simulink model "Rex_ProblemSet_4"  (R2020a)
settings: Solver=VariableStepAuto  StartTime=0.0  StopTime=10.0  RelTol=1e-3
libraries: commutil2 x4
settings Model: Creator=bayntuna  LastModifiedBy=23RexL

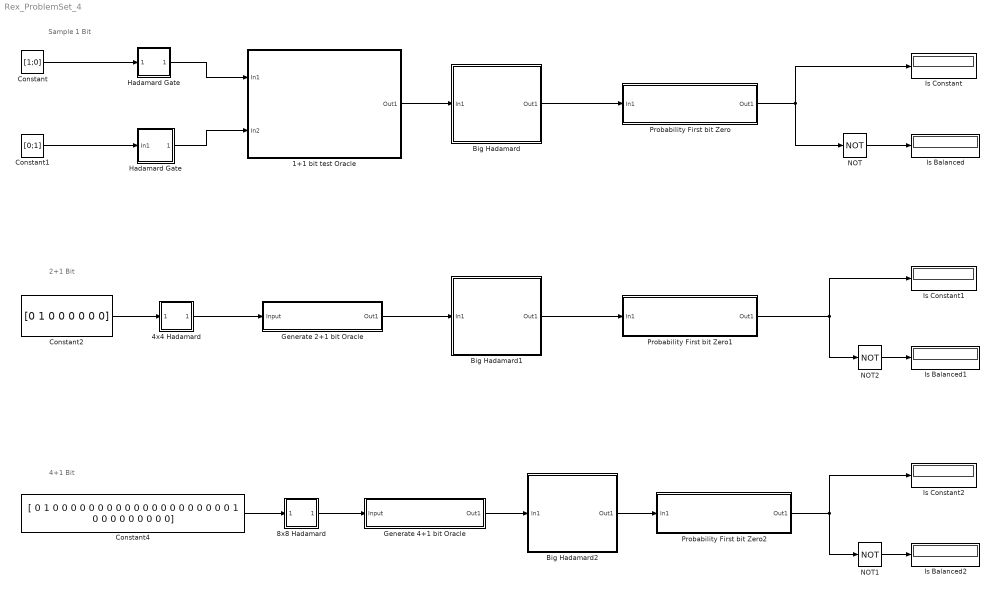
== system Rex_ProblemSet_4 ==
  note: 4+1 Bit
  note: 2+1 Bit
  note: Sample 1 Bit
  1+1 bit test Oracle : Subsystem
  4x4 Hadamard : Subsystem
  8x8 Hadamard : Subsystem
  Big Hadamard : Subsystem
  Big Hadamard1 : Subsystem
  Big Hadamard2 : Subsystem
  Constant : Constant  Value=[1;0]
  Constant1 : Constant  Value=[0;1]
  Constant2 : Constant  Value=[0 1 0 0 0 0 0 0]
  Constant4 : Constant  Value=[ 0 1 0 0 0 0 0 0 0 0 0 0 0 0 0 0 0 0 0 0 0 0 1 0 0 0 0 0 0 0 0 0]
  Generate 2+1 bit Oracle : Subsystem
  Generate 4+1 bit Oracle : Subsystem
  Hadamard Gate : Subsystem
  "Hadamard Gate " : Subsystem
  Is Balanced : Display
  Is Balanced1 : Display
  Is Balanced2 : Display
  Is Constant : Display
  Is Constant1 : Display
  Is Constant2 : Display
  NOT : Logic  Operator=NOT  IconShape=distinctive  AllPortsSameDT=off  OutDataTypeStr=boolean
  NOT1 : Logic  Operator=NOT  IconShape=distinctive  AllPortsSameDT=off  OutDataTypeStr=boolean
  NOT2 : Logic  Operator=NOT  IconShape=distinctive  AllPortsSameDT=off  OutDataTypeStr=boolean
  Probability First bit Zero : Subsystem
  Probability First bit Zero1 : Subsystem
  Probability First bit Zero2 : Subsystem
  wires:
  Constant/1 -> "Hadamard Gate "/1(In1)
  Constant1/1 -> Hadamard Gate/1(In1)
  "Hadamard Gate "/1(Out1) -> 1+1 bit test Oracle/1(In1)
  Hadamard Gate/1(Out1) -> 1+1 bit test Oracle/2(In2)
  1+1 bit test Oracle/1(Out1) -> Big Hadamard/1(In1)
  Big Hadamard/1(Out1) -> Probability First bit Zero/1(In1)
  Probability First bit Zero/1(Out1) -> Is Constant/1, NOT/1
  NOT/1 -> Is Balanced/1
  Generate 2+1 bit Oracle/1(Out1) -> Big Hadamard1/1(In1)
  NOT2/1 -> Is Balanced1/1
  Probability First bit Zero1/1(Out1) -> Is Constant1/1, NOT2/1
  Big Hadamard1/1(Out1) -> Probability First bit Zero1/1(In1)
  4x4 Hadamard/1(Input) -> Generate 2+1 bit Oracle/1(Input)
  Constant2/1 -> 4x4 Hadamard/1(In1)
  Constant4/1 -> 8x8 Hadamard/1(In1)
  8x8 Hadamard/1(Input) -> Generate 4+1 bit Oracle/1(Input)
  Generate 4+1 bit Oracle/1(Out1) -> Big Hadamard2/1(In1)
  Probability First bit Zero2/1(Out1) -> Is Constant2/1, NOT1/1
  NOT1/1 -> Is Balanced2/1
  Big Hadamard2/1(Out1) -> Probability First bit Zero2/1(In1)

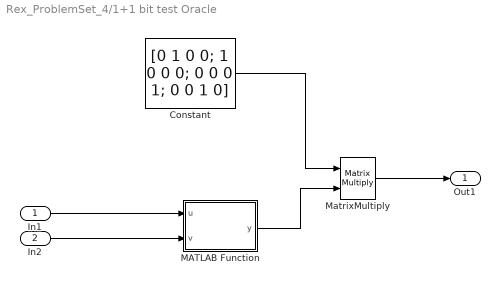
== system Rex_ProblemSet_4/1+1 bit test Oracle ==
  In1 : Inport
  In2 : Inport  Port=2
  Constant : Constant  Value=[0 1 0 0; 1 0 0 0; 0 0 0 1; 0 0 1 0]
  MATLAB Function : MATLAB Function  TreatAsAtomicUnit=on
  MatrixMultiply : Product  Multiplication=Matrix(*)
  Out1 : Outport
  wires:
  MatrixMultiply/1 -> Out1/1
  MATLAB Function/1(y) -> MatrixMultiply/2
  Constant/1 -> MatrixMultiply/1
  In1/1 -> MATLAB Function/1(u)
  In2/1 -> MATLAB Function/2(v)

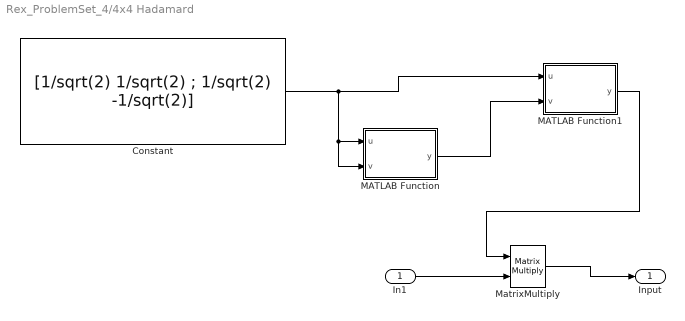
== system Rex_ProblemSet_4/4x4 Hadamard ==
  In1 : Inport
  Constant : Constant  Value=[1/sqrt(2) 1/sqrt(2) ; 1/sqrt(2) -1/sqrt(2)]
  MATLAB Function : MATLAB Function  TreatAsAtomicUnit=on
  MATLAB Function1 : MATLAB Function  TreatAsAtomicUnit=on
  MatrixMultiply : Product  Multiplication=Matrix(*)
  Input : Outport
  wires:
  MatrixMultiply/1 -> Input/1
  In1/1 -> MatrixMultiply/2
  Constant/1 -> MATLAB Function/2(v), MATLAB Function/1(u), MATLAB Function1/1(u)
  MATLAB Function/1(y) -> MATLAB Function1/2(v)
  MATLAB Function1/1(y) -> MatrixMultiply/1

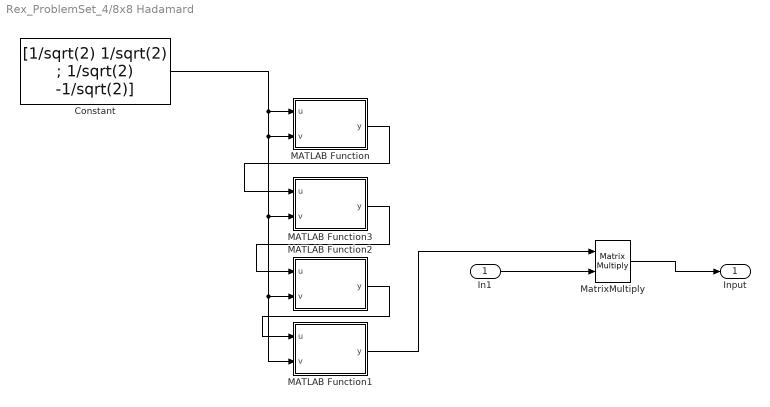
== system Rex_ProblemSet_4/8x8 Hadamard ==
  In1 : Inport
  Constant : Constant  Value=[1/sqrt(2) 1/sqrt(2) ; 1/sqrt(2) -1/sqrt(2)]
  MATLAB Function : MATLAB Function  TreatAsAtomicUnit=on
  MATLAB Function1 : MATLAB Function  TreatAsAtomicUnit=on
  MATLAB Function2 : MATLAB Function  TreatAsAtomicUnit=on
  MATLAB Function3 : MATLAB Function  TreatAsAtomicUnit=on
  MatrixMultiply : Product  Multiplication=Matrix(*)
  Input : Outport
  wires:
  MatrixMultiply/1 -> Input/1
  In1/1 -> MatrixMultiply/2
  Constant/1 -> MATLAB Function1/2(v), MATLAB Function2/2(v), MATLAB Function3/2(v), MATLAB Function/2(v), MATLAB Function/1(u)
  MATLAB Function1/1(y) -> MatrixMultiply/1
  MATLAB Function/1(y) -> MATLAB Function3/1(u)
  MATLAB Function3/1(y) -> MATLAB Function2/1(u)
  MATLAB Function2/1(y) -> MATLAB Function1/1(u)

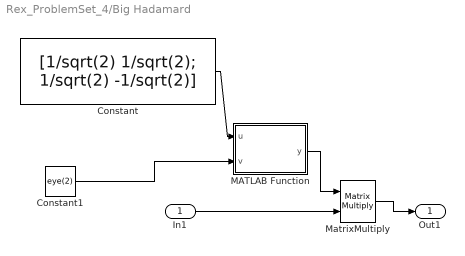
== system Rex_ProblemSet_4/Big Hadamard ==
  In1 : Inport
  Constant : Constant  Value=[1/sqrt(2) 1/sqrt(2); 1/sqrt(2) -1/sqrt(2)]
  Constant1 : Constant  Value=eye(2)
  MATLAB Function : MATLAB Function  TreatAsAtomicUnit=on
  MatrixMultiply : Product  Multiplication=Matrix(*)
  Out1 : Outport
  wires:
  In1/1 -> MatrixMultiply/2
  Constant1/1 -> MATLAB Function/2(v)
  Constant/1 -> MATLAB Function/1(u)
  MATLAB Function/1(y) -> MatrixMultiply/1
  MatrixMultiply/1 -> Out1/1

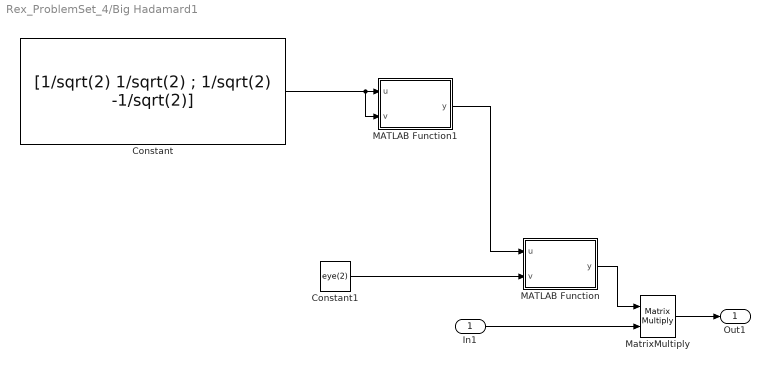
== system Rex_ProblemSet_4/Big Hadamard1 ==
  In1 : Inport
  Constant : Constant  Value=[1/sqrt(2) 1/sqrt(2) ; 1/sqrt(2) -1/sqrt(2)]
  Constant1 : Constant  Value=eye(2)
  MATLAB Function : MATLAB Function  TreatAsAtomicUnit=on
  MATLAB Function1 : MATLAB Function  TreatAsAtomicUnit=on
  MatrixMultiply : Product  Multiplication=Matrix(*)
  Out1 : Outport
  wires:
  In1/1 -> MatrixMultiply/2
  Constant1/1 -> MATLAB Function/2(v)
  MATLAB Function/1(y) -> MatrixMultiply/1
  MatrixMultiply/1 -> Out1/1
  Constant/1 -> MATLAB Function1/2(v), MATLAB Function1/1(u)
  MATLAB Function1/1(y) -> MATLAB Function/1(u)

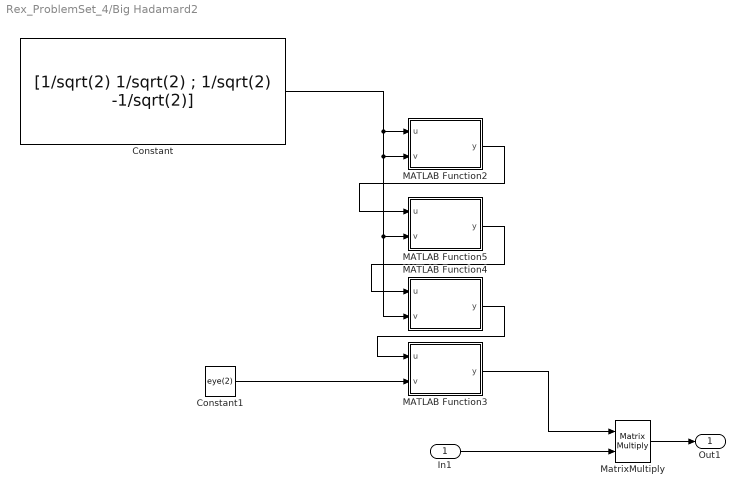
== system Rex_ProblemSet_4/Big Hadamard2 ==
  In1 : Inport
  Constant : Constant  Value=[1/sqrt(2) 1/sqrt(2) ; 1/sqrt(2) -1/sqrt(2)]
  Constant1 : Constant  Value=eye(2)
  MATLAB Function2 : MATLAB Function  TreatAsAtomicUnit=on
  MATLAB Function3 : MATLAB Function  TreatAsAtomicUnit=on
  MATLAB Function4 : MATLAB Function  TreatAsAtomicUnit=on
  MATLAB Function5 : MATLAB Function  TreatAsAtomicUnit=on
  MatrixMultiply : Product  Multiplication=Matrix(*)
  Out1 : Outport
  wires:
  In1/1 -> MatrixMultiply/2
  Constant1/1 -> MATLAB Function3/2(v)
  MATLAB Function3/1(y) -> MatrixMultiply/1
  MatrixMultiply/1 -> Out1/1
  MATLAB Function5/1(y) -> MATLAB Function4/1(u)
  MATLAB Function4/1(y) -> MATLAB Function3/1(u)
  MATLAB Function2/1(y) -> MATLAB Function5/1(u)
  Constant/1 -> MATLAB Function4/2(v), MATLAB Function5/2(v), MATLAB Function2/2(v), MATLAB Function2/1(u)

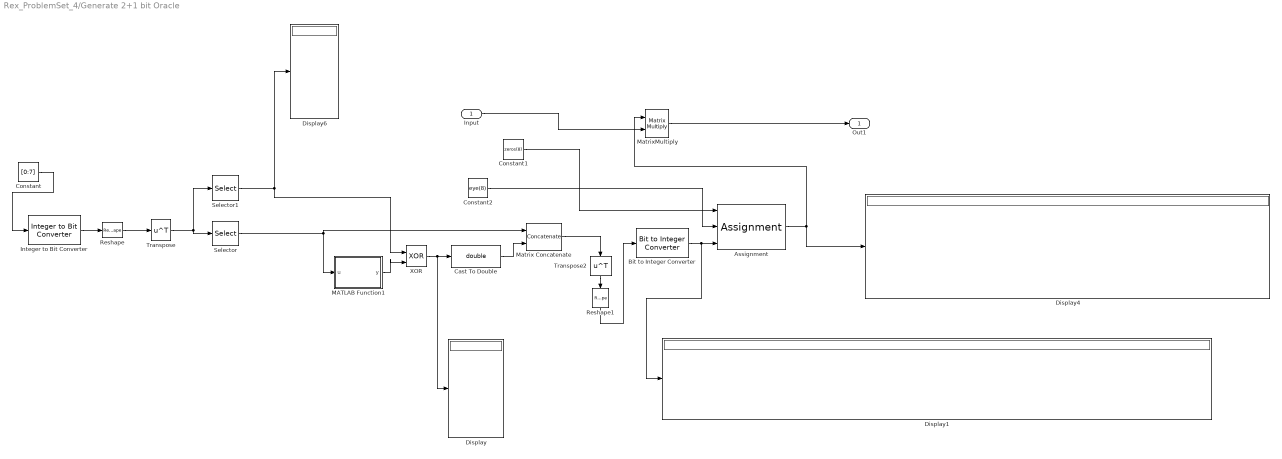
== system Rex_ProblemSet_4/Generate 2+1 bit Oracle ==
  Input : Inport
  Assignment : Assignment  NumberOfDimensions=2  IndexMode=Zero-based  DiagnosticForDimensions=Warning  IndexOptions=Assign all,Index vector (port)  Indices=1,1  OutputSizes=1,1
  Bit to Integer Converter : commutil2/Bit to Integer Converter  nbits=3  bitOrder=MSB first  signedOutputValues=Unsigned  outDtype=Inherit via internal rule  outDtypeSigned=Inherit via internal rule
  Cast To Double : DataTypeConversion  OutDataTypeStr=double
  Constant : Constant  Value=[0:7]
  Constant1 : Constant  Value=zeros(8)
  Constant2 : Constant  Value=eye(8)
  Display{,1,4,6} (4 alike) : Display
  Integer to Bit Converter : commutil2/Integer to Bit Converter  nbits=3  signedInputValues=Unsigned  bitOrder=MSB first  outDtype=Same as input
  MATLAB Function1 : MATLAB Function  TreatAsAtomicUnit=on
  Matrix Concatenate : Concatenate  Mode=Multidimensional array  ConcatenateDimension=2
  MatrixMultiply : Product  Multiplication=Matrix(*)
  Reshape : Reshape  OutputDimensionality=Customize  OutputDimensions=[3,8]
  Reshape1 : Reshape  OutputDimensionality=Column vector (2-D)  OutputDimensions=[1,8]
  Selector : Selector  NumberOfDimensions=2  InputPortWidth=3  IndexOptions=Select all,Index vector (dialog)  Indices=[2],[1 2]  OutputSizes=1,1
  Selector1 : Selector  NumberOfDimensions=2  InputPortWidth=3  IndexOptions=Select all,Index vector (dialog)  Indices=[1 3],3  OutputSizes=1,1
  Transpose : Math  Operator=transpose  SaturateOnIntegerOverflow=on
  Transpose2 : Math  Operator=transpose  SaturateOnIntegerOverflow=on
  XOR : Logic  Operator=XOR  IconShape=distinctive  AllPortsSameDT=off  OutDataTypeStr=boolean
  Out1 : Outport
  wires:
  Assignment/1 -> Display4/1, MatrixMultiply/1
  Selector/1 -> Matrix Concatenate/1, MATLAB Function1/1(u)
  Matrix Concatenate/1 -> Transpose2/1
  Transpose/1 -> Selector/1, Selector1/1
  XOR/1 -> Display/1, Cast To Double/1
  Constant/1 -> Integer to Bit Converter/1
  Constant2/1 -> Assignment/2
  Reshape1/1 -> Bit to Integer Converter/1
  Transpose2/1 -> Reshape1/1
  Integer to Bit Converter/1 -> Reshape/1
  Cast To Double/1 -> Matrix Concatenate/2
  Selector1/1 -> XOR/1, Display6/1
  Reshape/1 -> Transpose/1
  MATLAB Function1/1(y) -> XOR/2
  Constant1/1 -> Assignment/1
  Bit to Integer Converter/1 -> Display1/1, Assignment/3
  Input/1 -> MatrixMultiply/2
  MatrixMultiply/1 -> Out1/1

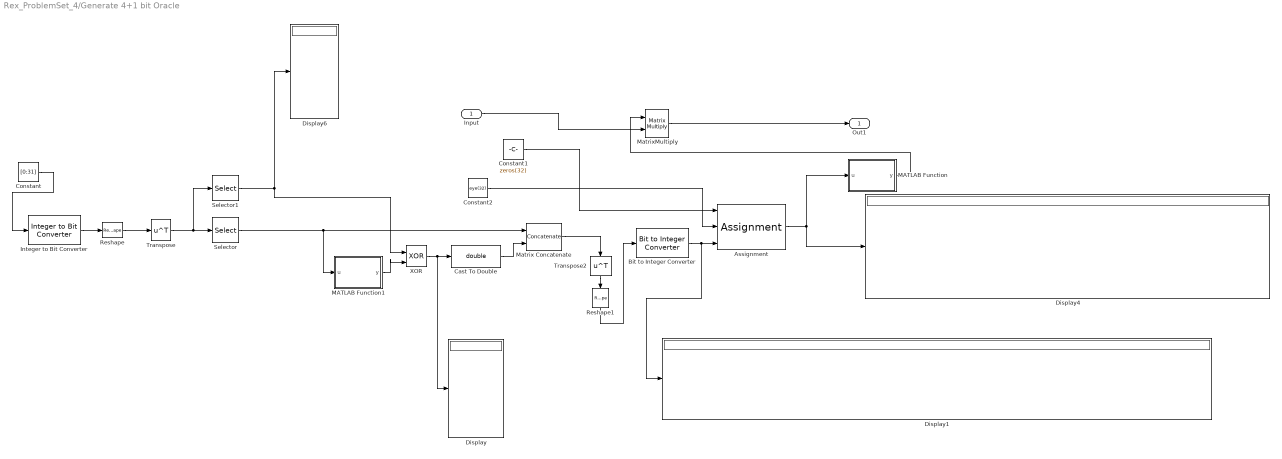
== system Rex_ProblemSet_4/Generate 4+1 bit Oracle ==
  Input : Inport
  Assignment : Assignment  NumberOfDimensions=2  IndexMode=Zero-based  DiagnosticForDimensions=Warning  IndexOptions=Assign all,Index vector (port)  Indices=1,1  OutputSizes=1,1
  Bit to Integer Converter : commutil2/Bit to Integer Converter  nbits=5  bitOrder=MSB first  signedOutputValues=Unsigned  outDtype=Inherit via internal rule  outDtypeSigned=Inherit via internal rule
  Cast To Double : DataTypeConversion  OutDataTypeStr=double
  Constant : Constant  Value=[0:31]
  Constant1 : Constant  Value=zeros(32)
  Constant2 : Constant  Value=eye(32)
  Display{,1,4,6} (4 alike) : Display
  Integer to Bit Converter : commutil2/Integer to Bit Converter  nbits=5  signedInputValues=Unsigned  bitOrder=MSB first  outDtype=Same as input
  MATLAB Function : MATLAB Function  TreatAsAtomicUnit=on
  MATLAB Function1 : MATLAB Function  TreatAsAtomicUnit=on
  Matrix Concatenate : Concatenate  Mode=Multidimensional array  ConcatenateDimension=2
  MatrixMultiply : Product  Multiplication=Matrix(*)
  Reshape : Reshape  OutputDimensionality=Customize  OutputDimensions=[5,32]
  Reshape1 : Reshape  OutputDimensionality=Column vector (2-D)  OutputDimensions=[1,8]
  Selector : Selector  NumberOfDimensions=2  InputPortWidth=3  IndexOptions=Select all,Index vector (dialog)  Indices=[2],[1 2 3 4]  OutputSizes=1,1
  Selector1 : Selector  NumberOfDimensions=2  InputPortWidth=3  IndexOptions=Select all,Index vector (dialog)  Indices=[1 3],5  OutputSizes=1,1
  Transpose : Math  Operator=transpose  SaturateOnIntegerOverflow=on
  Transpose2 : Math  Operator=transpose  SaturateOnIntegerOverflow=on
  XOR : Logic  Operator=XOR  IconShape=distinctive  AllPortsSameDT=off  OutDataTypeStr=boolean
  Out1 : Outport
  wires:
  Assignment/1 -> Display4/1, MATLAB Function/1(u)
  Selector/1 -> MATLAB Function1/1(u), Matrix Concatenate/1
  Matrix Concatenate/1 -> Transpose2/1
  XOR/1 -> Display/1, Cast To Double/1
  Constant/1 -> Integer to Bit Converter/1
  Constant2/1 -> Assignment/2
  Reshape1/1 -> Bit to Integer Converter/1
  Transpose2/1 -> Reshape1/1
  Integer to Bit Converter/1 -> Reshape/1
  Cast To Double/1 -> Matrix Concatenate/2
  Selector1/1 -> XOR/1, Display6/1
  Reshape/1 -> Transpose/1
  MATLAB Function1/1(y) -> XOR/2
  Constant1/1 -> Assignment/1
  Bit to Integer Converter/1 -> Display1/1, Assignment/3
  Input/1 -> MatrixMultiply/2
  MatrixMultiply/1 -> Out1/1
  Transpose/1 -> Selector/1, Selector1/1
  MATLAB Function/1(y) -> MatrixMultiply/1

== system Rex_ProblemSet_4/Hadamard Gate ==
  In1 : Inport
  Constant : Constant  Value=[1/sqrt(2) 1/sqrt(2); 1/sqrt(2) -1/sqrt(2)]
  MatrixMultiply : Product  Multiplication=Matrix(*)
  Out1 : Outport
  wires:
  MatrixMultiply/1 -> Out1/1
  In1/1 -> MatrixMultiply/2
  Constant/1 -> MatrixMultiply/1

== system Rex_ProblemSet_4/Hadamard Gate  ==
  In1 : Inport
  Constant : Constant  Value=[1/sqrt(2) 1/sqrt(2); 1/sqrt(2) -1/sqrt(2)]
  MatrixMultiply : Product  Multiplication=Matrix(*)
  Out1 : Outport
  wires:
  MatrixMultiply/1 -> Out1/1
  In1/1 -> MatrixMultiply/2
  Constant/1 -> MatrixMultiply/1

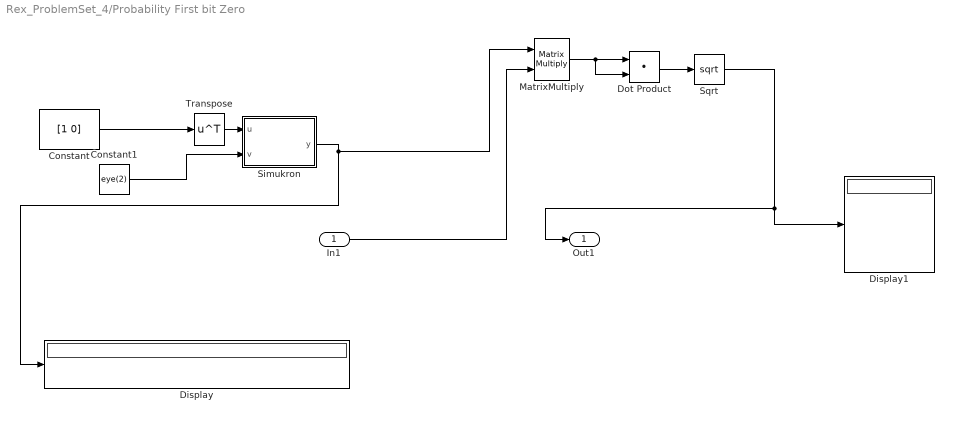
== system Rex_ProblemSet_4/Probability First bit Zero ==
  In1 : Inport
  Constant : Constant  Value=[1 0]
  Constant1 : Constant  Value=eye(2)
  Display : Display
  Display1 : Display
  Dot Product : DotProduct  InputSameDT=on  OutDataTypeStr=Inherit: Inherit via internal rule
  MatrixMultiply : Product  Multiplication=Matrix(*)
  Simukron : MATLAB Function  TreatAsAtomicUnit=on
  Sqrt : Sqrt  SaturateOnIntegerOverflow=on
  Transpose : Math  Operator=transpose  SaturateOnIntegerOverflow=on
  Out1 : Outport
  wires:
  Constant1/1 -> Simukron/2(v)
  Simukron/1(y) -> Display/1, MatrixMultiply/1
  Constant/1 -> Transpose/1
  Transpose/1 -> Simukron/1(u)
  In1/1 -> MatrixMultiply/2
  MatrixMultiply/1 -> Dot Product/2, Dot Product/1
  Sqrt/1 -> Out1/1, Display1/1
  Dot Product/1 -> Sqrt/1

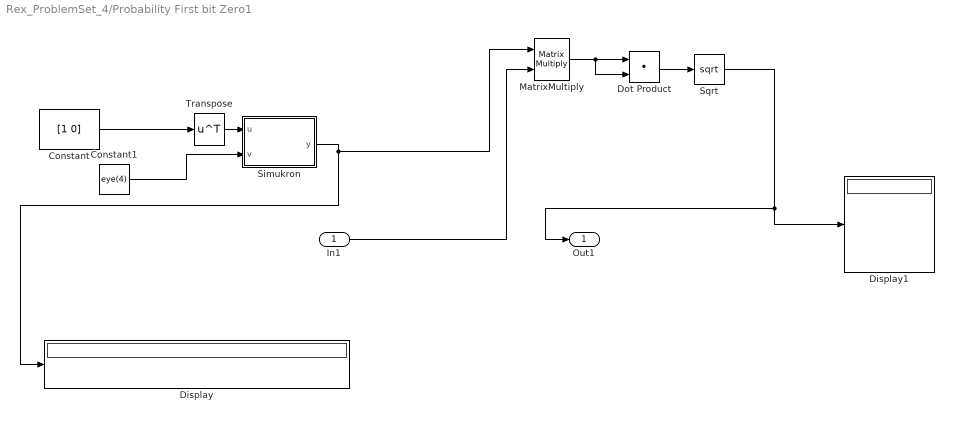
== system Rex_ProblemSet_4/Probability First bit Zero1 ==
  In1 : Inport
  Constant : Constant  Value=[1 0]
  Constant1 : Constant  Value=eye(4)
  Display : Display
  Display1 : Display
  Dot Product : DotProduct  InputSameDT=on  OutDataTypeStr=Inherit: Inherit via internal rule
  MatrixMultiply : Product  Multiplication=Matrix(*)
  Simukron : MATLAB Function  TreatAsAtomicUnit=on
  Sqrt : Sqrt  SaturateOnIntegerOverflow=on
  Transpose : Math  Operator=transpose  SaturateOnIntegerOverflow=on
  Out1 : Outport
  wires:
  Constant1/1 -> Simukron/2(v)
  Simukron/1(y) -> Display/1, MatrixMultiply/1
  Constant/1 -> Transpose/1
  Transpose/1 -> Simukron/1(u)
  In1/1 -> MatrixMultiply/2
  MatrixMultiply/1 -> Dot Product/2, Dot Product/1
  Sqrt/1 -> Out1/1, Display1/1
  Dot Product/1 -> Sqrt/1

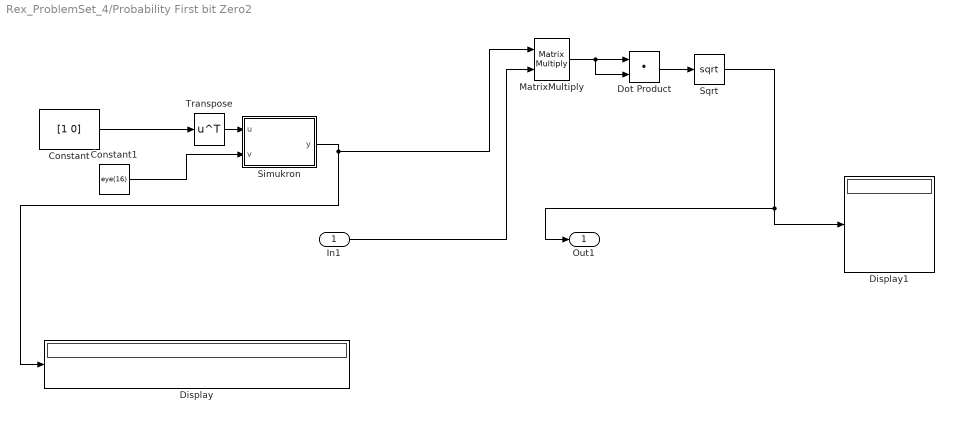
== system Rex_ProblemSet_4/Probability First bit Zero2 ==
  In1 : Inport
  Constant : Constant  Value=[1 0]
  Constant1 : Constant  Value=eye(16)
  Display : Display
  Display1 : Display
  Dot Product : DotProduct  InputSameDT=on  OutDataTypeStr=Inherit: Inherit via internal rule
  MatrixMultiply : Product  Multiplication=Matrix(*)
  Simukron : MATLAB Function  TreatAsAtomicUnit=on
  Sqrt : Sqrt  SaturateOnIntegerOverflow=on
  Transpose : Math  Operator=transpose  SaturateOnIntegerOverflow=on
  Out1 : Outport
  wires:
  Constant1/1 -> Simukron/2(v)
  Simukron/1(y) -> Display/1, MatrixMultiply/1
  Constant/1 -> Transpose/1
  Transpose/1 -> Simukron/1(u)
  In1/1 -> MatrixMultiply/2
  MatrixMultiply/1 -> Dot Product/2, Dot Product/1
  Sqrt/1 -> Out1/1, Display1/1
  Dot Product/1 -> Sqrt/1

== matlab function Rex_ProblemSet_4/8x8 Hadamard/MATLAB Function3 ==
  data: u input; y output; v input
function y = fcn(u, v)

y = kron(u,v);
end

== matlab function Rex_ProblemSet_4/Generate 4+1 bit Oracle/MATLAB Function1 ==
  data: u input; y output
function y = fcn(u)
m = size(u,1);
y = ones(m,1);
end

== matlab function Rex_ProblemSet_4/Probability First bit Zero2/Simukron ==
  data: u input; y output; v input
function y = fcn(u,v)
y = kron(u,v);
end

== matlab function Rex_ProblemSet_4/Big Hadamard2/MATLAB Function2 ==
  data: u input; y output; v input
function y = fcn(u,v)

y = kron(u,v);
end

== matlab function Rex_ProblemSet_4/Big Hadamard2/MATLAB Function3 ==
  data: u input; y output; v input
function y = fcn(u, v)

y = kron(u,v);
end

== matlab function Rex_ProblemSet_4/Big Hadamard2/MATLAB Function4 ==
  data: u input; y output; v input
function y = fcn(u, v)

y = kron(u,v);
end

== matlab function Rex_ProblemSet_4/Big Hadamard2/MATLAB Function5 ==
  data: u input; y output; v input
function y = fcn(u, v)

y = kron(u,v);
end

== matlab function Rex_ProblemSet_4/Generate 4+1 bit Oracle/MATLAB Function ==
  data: u input; y output
function y = fcn(u)

y = u - 1;

== matlab function Rex_ProblemSet_4/1+1 bit test Oracle/MATLAB Function ==
  data: u input; y output; v input
function y = fcn(u,v)

y = kron(u,v);
end

== matlab function Rex_ProblemSet_4/Probability First bit Zero/Simukron ==
  data: u input; y output; v input
function y = fcn(u,v)
y = kron(u,v);
end

== matlab function Rex_ProblemSet_4/Generate 2+1 bit Oracle/MATLAB Function1 ==
  data: u input; y output
function y = fcn(u)
m = size(u,1);
y = ones(m,1);
end

== matlab function Rex_ProblemSet_4/Big Hadamard1/MATLAB Function ==
  data: u input; y output; v input
function y = fcn(u,v)

y = kron(u,v);
end

== matlab function Rex_ProblemSet_4/Probability First bit Zero1/Simukron ==
  data: u input; y output; v input
function y = fcn(u,v)
y = kron(u,v);
end

== matlab function Rex_ProblemSet_4/4x4 Hadamard/MATLAB Function1 ==
  data: u input; y output; v input
function y = fcn(u,v)

y = kron(u,v);
end

== matlab function Rex_ProblemSet_4/4x4 Hadamard/MATLAB Function ==
  data: u input; y output; v input
function y = fcn(u,v)

y = kron(u,v);
end

== matlab function Rex_ProblemSet_4/Big Hadamard1/MATLAB Function1 ==
  data: u input; y output; v input
function y = fcn(u,v)

y = kron(u,v);
end

== matlab function Rex_ProblemSet_4/8x8 Hadamard/MATLAB Function ==
  data: u input; y output; v input
function y = fcn(u,v)

y = kron(u,v);
end

== matlab function Rex_ProblemSet_4/8x8 Hadamard/MATLAB Function1 ==
  data: u input; y output; v input
function y = fcn(u, v)

y = kron(u,v);
end

== matlab function Rex_ProblemSet_4/Big Hadamard/MATLAB Function ==
  data: u input; y output; v input
function y = fcn(u,v)

y = kron(u,v);
end

== matlab function Rex_ProblemSet_4/8x8 Hadamard/MATLAB Function2 ==
  data: u input; y output; v input
function y = fcn(u, v)

y = kron(u,v);
end
